simulink model "FIRfilter6"  (R2020a)
settings: Solver=FixedStepAuto  StartTime=0.0  StopTime=10.0  FixedStep=0.2  RelTol=1e-3
settings Model: Creator=Anjali123  LastModifiedBy=Anjali123
settings DataIOCC: SaveOutput=off  SaveTime=off

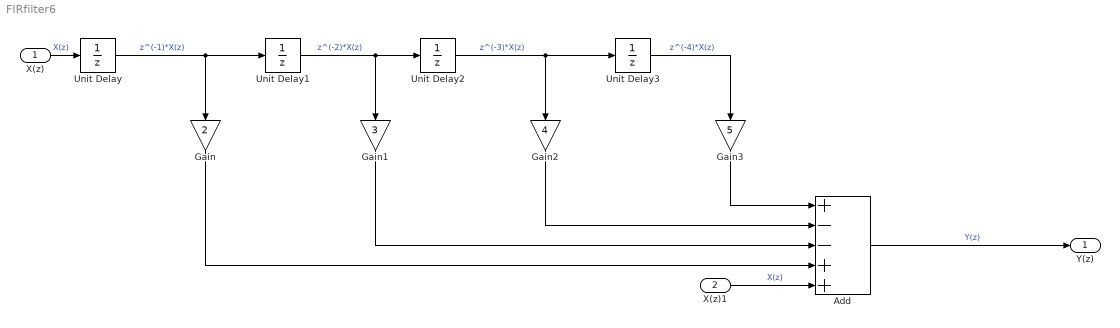
== system FIRfilter6 ==
  X(z) : Inport  OutDataTypeStr=double  PortDimensions=1  SampleTime=[0.20000000000000001,0]
  X(z)1 : Inport  Port=2  OutDataTypeStr=double  PortDimensions=1  SampleTime=[0.20000000000000001,0]
  Add : Sum  Inputs=+--++
  Gain : Gain  Gain=2
  Gain1 : Gain  Gain=3
  Gain2 : Gain  Gain=4
  Gain3 : Gain  Gain=5
  Unit Delay{,1..3} (4 alike) : UnitDelay  SampleTime=-1  HasFrameUpgradeWarning=on
  Y(z) : Outport  OutDataTypeStr=double  PortDimensions=1  SampleTime=[0.20000000000000001,0]
  wires:
  Gain3/1 -> Add/1
  Unit Delay/1 -> Gain/1, Unit Delay1/1  "z^(-1)*X(z)"
  Unit Delay1/1 -> Unit Delay2/1, Gain1/1  "z^(-2)*X(z)"
  Unit Delay2/1 -> Unit Delay3/1, Gain2/1  "z^(-3)*X(z)"
  Gain/1 -> Add/4
  Gain1/1 -> Add/3
  Unit Delay3/1 -> Gain3/1  "z^(-4)*X(z)"
  X(z)1/1 -> Add/5  "X(z)"
  Gain2/1 -> Add/2
  Add/1 -> Y(z)/1  "Y(z)"
  X(z)/1 -> Unit Delay/1  "X(z)"
